simulink model "active_vehicle_controller_functions"  (R2020a)
settings: Solver=ode4  StartTime=0.0  StopTime=inf  FixedStep=1e-3  RelTol=1e-3
InitFcn:
  | clear mex
undefined symbols (not defined in the file or in its folder): DiscIntNeverNeededParam, vicrt_initcallback, vicrt_initmexcallback, vicrt_inputfile, vicrt_simulationmanager
libraries: simulink x1
(part 1 of 6)
settings Model: Creator=mcava  LastModifiedBy=lucas
settings DataIOCC: LimitDataPoints=on  SaveFormat=Array  SignalLoggingSaveFormat=ModelDataLogs  ReturnWorkspaceOutputs=off  SignalLoggingName=sigsOut
settings OptimizationCC: ExpressionDepthLimit=2147483647  InitFltsAndDblsToZero=on  LifeSpan=inf
settings DebuggingCC: SignalInfNanChecking=warning  SaveWithParameterizedLinksMsg=none  UnderspecifiedInitializationDetection=Classic  MergeDetectMultiDrivingBlocksExec=none  SignalResolutionControl=TryResolveAllWithWarning  MultiTaskDSMMsg=warning  MultiTaskCondExecSysMsg=none  FcnCallInpInsideContextMsg=warning  StateNameClashWarn=warning  SFUnexpectedBacktrackingDiag=warning  SFNoUnconditionalDefaultTransitionDiag=warning  SFExecutionAtInitializationDiag=none  ArithmeticOperatorsInVariantConditions=warning
settings HardwareCC: ProdBitPerPointer=32  ProdBitPerSizeT=32  ProdBitPerPtrDiffT=32  ProdLargestAtomicFloat=None  ProdIntDivRoundTo=Undefined  ProdEndianess=Unspecified  ProdWordSize=32  ProdHWDeviceType=32-bit Generic  TargetBitPerPointer=64  TargetBitPerSizeT=64  TargetBitPerPtrDiffT=64  TargetLongLongMode=on  TargetIntDivRoundTo=Zero  TargetEndianess=LittleEndian  TargetWordSize=64  TargetHWDeviceType=MATLAB Host  ProdEqTarget=off
settings ModelReferenceCC: PropagateSignalLabelsOutOfModel=off
settings SFSimCC: SimUseLocalCustomCode=off  SimParseCustomCode=off  CustomCodeUndefinedFunction=UseInterfaceOnly
settings RTWCC: RTWVerbose=off  RTWUseLocalCustomCode=off
settings CodeAppCC: GenerateComments=off  SimulinkBlockComments=off
settings GRTTargetCC: TargetFcnLib=ansi_tfl_tmw.mat  TargetLangStandard=C89/C90 (ANSI)  CombineOutputUpdateFcns=off  GRTInterface=on
settings ConfigComp: CovMetricSettings=dw  CovHtmlReporting=on  CovSaveCumulativeToWorkspaceVar=on  CovSaveSingleToWorkspaceVar=on  CovExternalEMLEnable=off

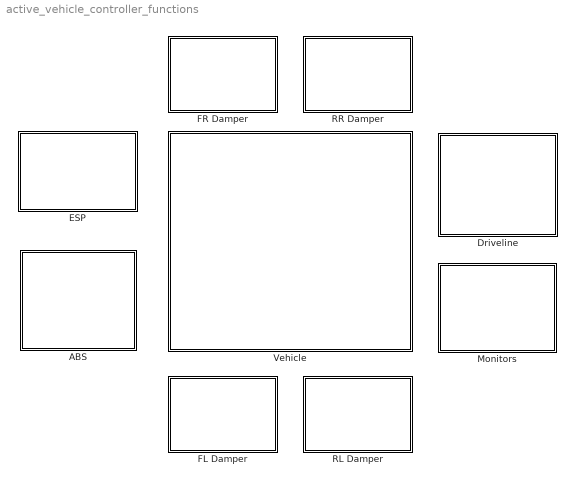
== system active_vehicle_controller_functions ==
  ABS : Subsystem  mask{ABSActive=on}
      mask prompts: ABSActive "Active"
      mask Display: image(imread('abs.jpg'))
  Driveline : Subsystem
      mask Display: image(imread('driveline.jpg'))
  ESP : Subsystem  mask(ESP Controller){ESPActive=on, WheelBase=2.838, SteeringRatio=(7.85/54)}
      mask prompts: ESPActive "Active"
      mask help:
      | Active toggle switches ESP On/Off
      | WheelBase and SteeringRatio parameters are used  to calculate theorical Vehicle Yaw Rate.
      mask Display: image(imread('esp.jpg'))
  FL Damper : Subsystem  mask{FLDamperActive=off}
      mask prompts: FLDamperActive "Active"
      mask Display: image(imread('damper.jpg'))
  FR Damper : Subsystem  mask{FRDamperActive=off}
      mask prompts: FRDamperActive "Active"
      mask Display: image(imread('damper.jpg'))
  Monitors : Subsystem
      mask Display: image(imread('monitors.jpg'))
  RL Damper : Subsystem  mask{RLDamperActive=off}
      mask prompts: RLDamperActive "Active"
      mask Display: image(imread('damper.jpg'))
  RR Damper : Subsystem  mask{RRDamperActive=off}
      mask prompts: RRDamperActive "Active"
      mask Display: image(imread('damper.jpg'))
  Vehicle : Subsystem
      mask Display: image(imread('vehicle.jpg'))

== system active_vehicle_controller_functions/ABS ==
  1st Order Lag L1 : TransferFcn  Denominator="[0.05  1]"
  1st Order Lag L2 : TransferFcn  Denominator="[0.05  1]"
  1st Order Lag R1 : TransferFcn  Denominator="[0.05  1]"
  1st Order Lag R2 : TransferFcn  Denominator="[0.05  1]"
  Brakes Already On? : Switch  Criteria=u2 > Threshold  SaturateOnIntegerOverflow=on
  Brakes Off : Constant  Value=0
  Brakes On : Constant
  Constant : Constant  Value=ABSActive
  Control Modes : Scope
  Demux : Demux
      settings: DisplayOption=none
  Memory : Memory  InitialCondition=[1,1,1,1]
  Mux : Mux
  NO ABS : Constant  Value=[1,1,1,1]
  Slip < Slip On? : Switch  Threshold=0.1  SaturateOnIntegerOverflow=on
  Slip > Slip Off? : Switch  Criteria=u2 > Threshold  Threshold=0.2  SaturateOnIntegerOverflow=on
  Slip Ratios : Product  Inputs=*/  SaturateOnIntegerOverflow=on  OutDataTypeStr=Inherit: Same as first input
  Slips : Scope
  Sum : Sum  Inputs=-+  SaturateOnIntegerOverflow=on  OutDataTypeStr=Inherit: Same as first input
  Vx > Vmin? : Switch  Criteria=u2 > Threshold  Threshold=5  SaturateOnIntegerOverflow=on
  Vx > Vmin?1 : Switch  Criteria=u2 > Threshold  SaturateOnIntegerOverflow=on
  tag scope: BrakesPressureGains=global
  wires:
  Sum/1 -> Slip Ratios/1
  [SprungMassCGVx] -> Slip Ratios/2, Sum/2, Vx > Vmin?/2
  Vx > Vmin?/1 -> Memory/1, Control Modes/1, Demux/1
  Slip > Slip Off?/1 -> Vx > Vmin?/1
  Brakes On/1 -> Brakes Already On?/1, Vx > Vmin?/3, Slip < Slip On?/3
  Brakes Off/1 -> Slip > Slip Off?/1, Brakes Already On?/3
  Slip Ratios/1 -> Slips/1, Slip > Slip Off?/2, Slip < Slip On?/2
  Slip < Slip On?/1 -> Slip > Slip Off?/3
  Memory/1 -> Brakes Already On?/2
  Brakes Already On?/1 -> Slip < Slip On?/1
  Demux/4 -> 1st Order Lag R2/1
  Demux/3 -> 1st Order Lag R1/1
  Demux/2 -> 1st Order Lag L2/1
  Demux/1 -> 1st Order Lag L1/1
  1st Order Lag L1/1 -> Mux/1
  1st Order Lag L2/1 -> Mux/2
  1st Order Lag R1/1 -> Mux/3
  1st Order Lag R2/1 -> Mux/4
  Mux/1 -> Vx > Vmin?1/1
  [TireTreadVx] -> Sum/1
  Constant/1 -> Vx > Vmin?1/2
  Vx > Vmin?1/1 -> [BrakesPressureGains]
  NO ABS/1 -> Vx > Vmin?1/3

== system active_vehicle_controller_functions/Driveline ==
  Clutch : Subsystem  mask{UserClutchActive=off}
      mask prompts: UserClutchActive "Active"
      mask Display: image(imread('clutch.jpg'))
  Engine : Subsystem  mask{UserEngineActive=off}
      mask prompts: UserEngineActive "Active"
      mask Display: image(imread('engine.jpg'))
  GearBox : Subsystem  mask{UserGearBoxActive=off}
      mask prompts: UserGearBoxActive "Active"
      mask Display: image(imread('gearbox.jpg'))
  Rear Differential : Subsystem  mask{RearDifferentialActive=off, DriveRatio=3.7}
      mask prompts: RearDifferentialActive "Active"; DriveRatio "Drive Ratio"
      mask Display: image(imread('differential.jpg'))

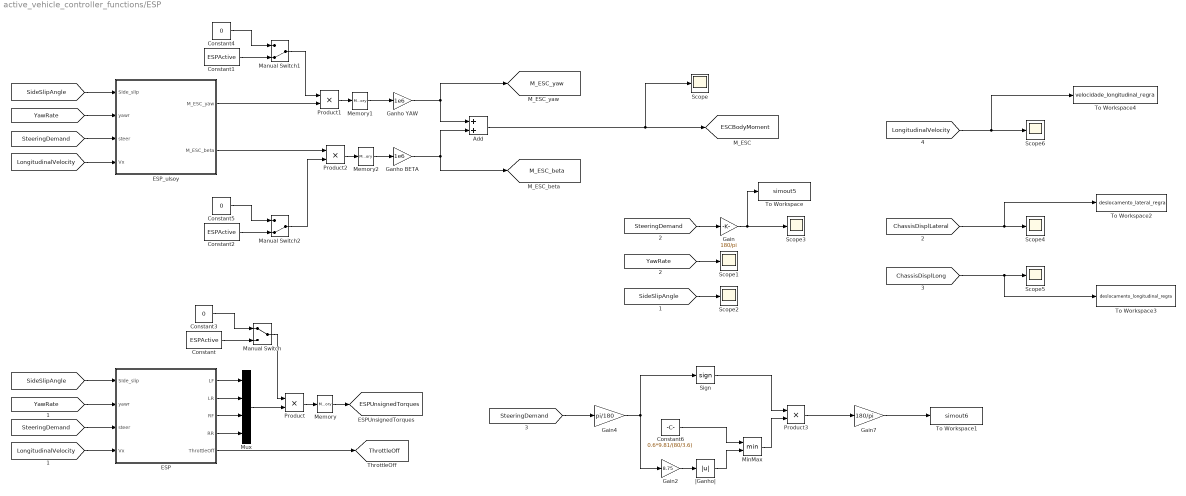
== system active_vehicle_controller_functions/ESP ==
  Add : Sum
  Constant : Constant  Value=ESPActive
  Constant1 : Constant  Value=ESPActive
  Constant2 : Constant  Value=ESPActive
  Constant3 : Constant  Value=0
  Constant4 : Constant  Value=0
  Constant5 : Constant  Value=0
  Constant6 : Constant  Value=0.6*9.81/(80/3.6)
  ESP : Subsystem  TreatAsAtomicUnit=on
  ESP_ulsoy : Subsystem  TreatAsAtomicUnit=on
  Gain : Gain  Gain=180/pi
  Gain2 : Gain  Gain=8.75
  Gain4 : Gain  Gain=pi/180
  Gain7 : Gain  Gain=180/pi
  Ganho BETA : Gain  Gain=1e6
  Ganho YAW : Gain  Gain=1e6
  Manual Switch : ManualSwitch
  Manual Switch1 : ManualSwitch  CurrentSetting=0
  Manual Switch2 : ManualSwitch  CurrentSetting=0
  Memory : Memory  InitialCondition=[0,0,0,0]
  Memory1 : Memory  InitialCondition=[0]
  Memory2 : Memory  InitialCondition=[0]
  MinMax : MinMax  Inputs=2
  Mux : Mux
  Product : Product  RndMeth=Zero  OutDataTypeStr=Inherit: Same as first input
  Product1 : Product  RndMeth=Zero  OutDataTypeStr=Inherit: Same as first input
  Product2 : Product  RndMeth=Zero  OutDataTypeStr=Inherit: Same as first input
  Product3 : Product
  Scope{,1..6} (7 alike) : Scope
  Sign : Signum
  To Workspace : ToWorkspace  VariableName=simout5  SaveFormat=Timeseries  SampleTime=-1
  To Workspace1 : ToWorkspace  VariableName=simout6  SaveFormat=Timeseries  SampleTime=-1
  To Workspace2 : ToWorkspace  VariableName=deslocamento_lateral_regra  SampleTime=-1
  To Workspace3 : ToWorkspace  VariableName=deslocamento_longitudinal_regra  SampleTime=-1
  To Workspace4 : ToWorkspace  VariableName=velocidade_longitudinal_regra  SaveFormat=Timeseries  SampleTime=-1
  |Ganho| : Abs
  tag scope: ESCBodyMoment=global, ESPUnsignedTorques=global, M_ESC_beta=global, M_ESC_yaw=global, ThrottleOff=global
  wires:
  [SideSlipAngle] -> ESP_ulsoy/1(SIde_slip)
  [LongitudinalVelocity] -> ESP_ulsoy/4(Vx)
  [YawRate] -> ESP_ulsoy/2("yawr ")
  [SteeringDemand] -> ESP_ulsoy/3(steer)
  Product1/1 -> Memory1/1
  Memory1/1 -> Ganho YAW/1
  ESP_ulsoy/1(M_ESC_yaw) -> Product1/2
  ESP/1(LF) -> Mux/1
  Mux/1 -> Product/2
  Memory/1 -> [ESPUnsignedTorques]
  [SteeringDemand] -> ESP/3(steer)
  ESP/4(RR) -> Mux/4
  ESP/2(LR) -> Mux/2
  [LongitudinalVelocity] -> ESP/4(Vx)
  [SideSlipAngle] -> ESP/1(SIde_slip)
  ESP/5(ThrottleOff) -> [ThrottleOff]
  Product/1 -> Memory/1
  ESP/3(RF) -> Mux/3
  [YawRate] -> ESP/2("yawr ")
  Memory2/1 -> Ganho BETA/1
  Product2/1 -> Memory2/1
  ESP_ulsoy/2(M_ESC_beta) -> Product2/1
  Add/1 -> [ESCBodyMoment], Scope/1
  Ganho YAW/1 -> [M_ESC_yaw], Add/1
  Ganho BETA/1 -> [M_ESC_beta], Add/2
  Manual Switch/1 -> Product/1
  Constant/1 -> Manual Switch/2
  Constant3/1 -> Manual Switch/1
  Constant4/1 -> Manual Switch1/1
  Constant1/1 -> Manual Switch1/2
  Manual Switch1/1 -> Product1/1
  Constant5/1 -> Manual Switch2/1
  Constant2/1 -> Manual Switch2/2
  Manual Switch2/1 -> Product2/2
  [YawRate] -> Scope1/1
  [SideSlipAngle] -> Scope2/1
  [SteeringDemand] -> Gain/1
  Gain/1 -> Scope3/1, To Workspace/1
  Gain4/1 -> Gain2/1, Sign/1
  |Ganho|/1 -> MinMax/2
  MinMax/1 -> Product3/2
  Constant6/1 -> MinMax/1
  [SteeringDemand] -> Gain4/1
  Sign/1 -> Product3/1
  Gain2/1 -> |Ganho|/1
  Gain7/1 -> To Workspace1/1
  Product3/1 -> Gain7/1
  [ChassisDisplLong] -> To Workspace3/1, Scope5/1
  [ChassisDisplLateral] -> Scope4/1, To Workspace2/1
  [LongitudinalVelocity] -> Scope6/1, To Workspace4/1

== system active_vehicle_controller_functions/FL Damper ==
  "C " : Gain  Gain=4000  OutDataTypeStr=Inherit: Same as input  ParamDataTypeStr=Inherit: Same as input
  Constant : Constant  Value=FLDamperActive
  Data Type Conversion : DataTypeConversion
  DmpF Lookup : Lookup  InputValues=|  Table=|
      InputValues=|
      | [ -1.5800000e+000 -1.0200000e+000 -7.7000000e-001 -5.1000000e-001 -3.8000000e-001 -2.5000000e-001 -1.3000000e-001 -5.0000000e-002 -3.0000000e-002 -1.0000000e-002  0.0000000e+000  1.0000000e-002  3.0000000e-002  5.0000000e-002  1.3000000e-001  2.6000000e-001  3.8000000e-001  5.1000000e-001  7.8000000e-001  1.0400000e+000  1.6200000e+000	
      | ]
      Table=|
      | [ -3.2605700e+003 -2.6592520e+003 -2.3311553e+003 -1.9825529e+003 -1.7569865e+003 -1.5314201e+003 -1.2853477e+003 -8.9573310e+002 -7.0015000e+002 -3.9192000e+002  0.0000000e+000  1.7058070e+002  4.3715920e+002  6.6272540e+002  1.0113279e+003  1.4419546e+003  1.6470150e+003  1.7905570e+003  2.1107987e+003  2.4057380e+003  3.1155941e+003	
      | ]
  Gain : Gain  Gain=1.2  OutDataTypeStr=Inherit: Same as input  ParamDataTypeStr=Inherit: Same as input
  Lin/Spline switch : ManualSwitch
  Logical Operator : Logic  Operator=NOT  AllPortsSameDT=off  OutDataTypeStr=boolean
  Memory : Memory
  Minus1 : UnaryMinus
  Minus2 : UnaryMinus
  Product : Product  RndMeth=Zero  OutDataTypeStr=Inherit: Same as first input
  Product1 : Product  RndMeth=Zero  OutDataTypeStr=Inherit: Same as first input
  Vx Lookup : Lookup  InputValues=|  Table=|
      InputValues=|
      | [ -5e-2 -1e-2 -5e-3 0 5e-3 1e-2 5e-2
      | ]
      Table=|
      | [ 1 1 1 0.2 1 1 1
      | ]
  tag scope: FLDamperForce=global, InternalFLDamperActive=global
  wires:
  Product/1 -> [FLDamperForce]
  Memory/1 -> Product/1
  Lin/Spline switch/1 -> Memory/1
  [FLDamperVelocity] -> Minus2/1, "C "/1
  Minus2/1 -> DmpF Lookup/1
  DmpF Lookup/1 -> Minus1/1
  "C "/1 -> Lin/Spline switch/2
  Minus1/1 -> Product1/2
  Product1/1 -> Lin/Spline switch/1
  Vx Lookup/1 -> Gain/1
  Gain/1 -> Product1/1
  [VerticalVelocity] -> Vx Lookup/1
  Data Type Conversion/1 -> [InternalFLDamperActive]
  Constant/1 -> Product/2, Logical Operator/1
  Logical Operator/1 -> Data Type Conversion/1

== system active_vehicle_controller_functions/FR Damper ==
  "C " : Gain  Gain=4000  OutDataTypeStr=Inherit: Same as input  ParamDataTypeStr=Inherit: Same as input
  Constant : Constant  Value=FRDamperActive
  Data Type Conversion : DataTypeConversion
  DmpF Lookup : Lookup  InputValues=|  Table=|
      InputValues=|
      | [ -1.5800000e+000 -1.0200000e+000 -7.7000000e-001 -5.1000000e-001 -3.8000000e-001 -2.5000000e-001 -1.3000000e-001 -5.0000000e-002 -3.0000000e-002 -1.0000000e-002  0.0000000e+000  1.0000000e-002  3.0000000e-002  5.0000000e-002  1.3000000e-001  2.6000000e-001  3.8000000e-001  5.1000000e-001  7.8000000e-001  1.0400000e+000  1.6200000e+000	
      | ]
      Table=|
      | [ -3.2605700e+003 -2.6592520e+003 -2.3311553e+003 -1.9825529e+003 -1.7569865e+003 -1.5314201e+003 -1.2853477e+003 -8.9573310e+002 -7.0015000e+002 -3.9192000e+002  0.0000000e+000  1.7058070e+002  4.3715920e+002  6.6272540e+002  1.0113279e+003  1.4419546e+003  1.6470150e+003  1.7905570e+003  2.1107987e+003  2.4057380e+003  3.1155941e+003	
      | ]
  Gain : Gain  Gain=1.2  OutDataTypeStr=Inherit: Same as input  ParamDataTypeStr=Inherit: Same as input
  Lin/Spline switch : ManualSwitch
  Logical Operator : Logic  Operator=NOT  AllPortsSameDT=off  OutDataTypeStr=boolean
  Memory : Memory
  Minus1 : UnaryMinus
  Minus2 : UnaryMinus
  Product : Product  RndMeth=Zero  OutDataTypeStr=Inherit: Same as first input
  Product1 : Product  RndMeth=Zero  OutDataTypeStr=Inherit: Same as first input
  Vx Lookup : Lookup  InputValues=|  Table=|
      InputValues=|
      | [ -5e-2 -1e-2 -5e-3 0 5e-3 1e-2 5e-2
      | ]
      Table=|
      | [ 1 1 1 0.2 1 1 1
      | ]
  tag scope: FRDamperForce=global, InternalFRDamperActive=global
  wires:
  Data Type Conversion/1 -> [InternalFRDamperActive]
  Memory/1 -> Product/1
  Product/1 -> [FRDamperForce]
  Lin/Spline switch/1 -> Memory/1
  [FRDamperVelocity] -> Minus2/1, "C "/1
  Minus2/1 -> DmpF Lookup/1
  DmpF Lookup/1 -> Minus1/1
  "C "/1 -> Lin/Spline switch/2
  Minus1/1 -> Product1/2
  Product1/1 -> Lin/Spline switch/1
  Vx Lookup/1 -> Gain/1
  Gain/1 -> Product1/1
  [VerticalVelocity] -> Vx Lookup/1
  Constant/1 -> Product/2, Logical Operator/1
  Logical Operator/1 -> Data Type Conversion/1

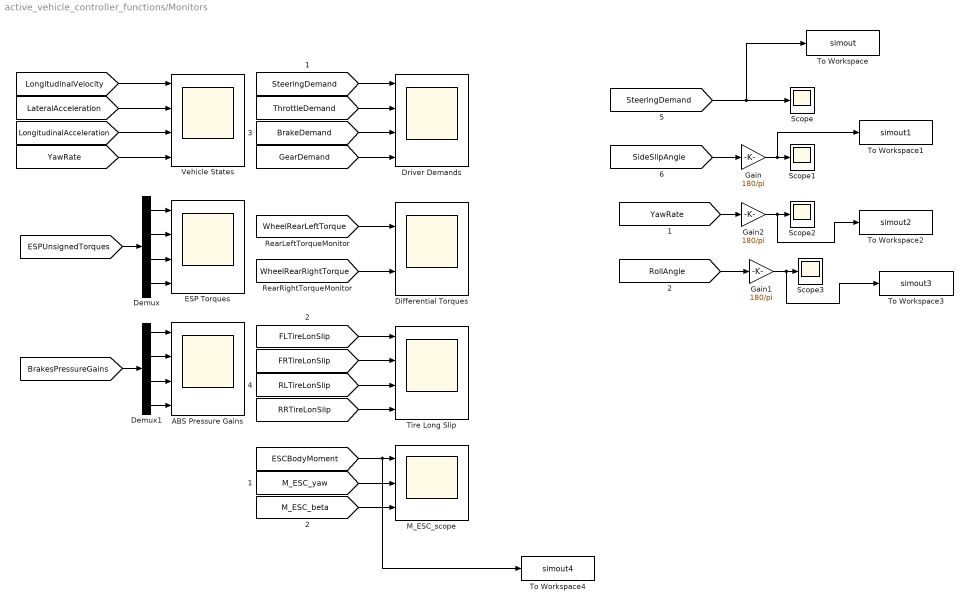
== system active_vehicle_controller_functions/Monitors ==
  ABS Pressure Gains : Scope  NumInputPorts=4
  Demux : Demux
  Demux1 : Demux
  Differential Torques : Scope  NumInputPorts=2
  Driver Demands : Scope  NumInputPorts=4
  ESP Torques : Scope  NumInputPorts=4
  Gain : Gain  Gain=180/pi
  Gain1 : Gain  Gain=180/pi
  Gain2 : Gain  Gain=180/pi
  M_ESC_scope : Scope  NumInputPorts=3
  Scope{,1..3} (4 alike) : Scope
  Tire Long Slip : Scope  NumInputPorts=4
  To Workspace : ToWorkspace  VariableName=simout  SaveFormat=Timeseries  SampleTime=-1
  To Workspace1 : ToWorkspace  VariableName=simout1  SaveFormat=Timeseries  SampleTime=-1
  To Workspace2 : ToWorkspace  VariableName=simout2  SaveFormat=Timeseries  SampleTime=-1
  To Workspace3 : ToWorkspace  VariableName=simout3  SaveFormat=Timeseries  SampleTime=-1
  To Workspace4 : ToWorkspace  VariableName=simout4  SaveFormat=Timeseries  SampleTime=-1
  Vehicle States : Scope  NumInputPorts=4
  wires:
  [LongitudinalVelocity] -> Vehicle States/1
  [LateralAcceleration] -> Vehicle States/2
  [LongitudinalAcceleration] -> Vehicle States/3
  [YawRate] -> Vehicle States/4
  [SteeringDemand] -> Driver Demands/1
  [ThrottleDemand] -> Driver Demands/2
  [BrakeDemand] -> Driver Demands/3
  [GearDemand] -> Driver Demands/4
  [ESPUnsignedTorques] -> Demux/1
  Demux/1 -> ESP Torques/1
  Demux/2 -> ESP Torques/2
  Demux/3 -> ESP Torques/3
  Demux/4 -> ESP Torques/4
  Demux1/1 -> ABS Pressure Gains/1
  Demux1/2 -> ABS Pressure Gains/2
  Demux1/3 -> ABS Pressure Gains/3
  Demux1/4 -> ABS Pressure Gains/4
  [BrakesPressureGains] -> Demux1/1
  [FLTireLonSlip] -> Tire Long Slip/1
  [FRTireLonSlip] -> Tire Long Slip/2
  [RLTireLonSlip] -> Tire Long Slip/3
  [RRTireLonSlip] -> Tire Long Slip/4
  [WheelRearLeftTorque] -> Differential Torques/1
  [WheelRearRightTorque] -> Differential Torques/2
  [ESCBodyMoment] -> To Workspace4/1, M_ESC_scope/1
  [M_ESC_yaw] -> M_ESC_scope/2
  [M_ESC_beta] -> M_ESC_scope/3
  [SteeringDemand] -> Scope/1, To Workspace/1
  [RollAngle] -> Gain1/1
  Gain1/1 -> To Workspace3/1, Scope3/1
  [YawRate] -> Gain2/1
  Gain2/1 -> To Workspace2/1, Scope2/1
  Gain/1 -> To Workspace1/1, Scope1/1
  [SideSlipAngle] -> Gain/1

== system active_vehicle_controller_functions/RL Damper ==
  "C " : Gain  Gain=4000  OutDataTypeStr=Inherit: Same as input  ParamDataTypeStr=Inherit: Same as input
  Constant : Constant  Value=RLDamperActive
  Data Type Conversion : DataTypeConversion
  DmpF Lookup : Lookup  InputValues=|  Table=|
      InputValues=|
      | [ -1.5800000e+000 -1.0200000e+000 -7.7000000e-001 -5.1000000e-001 -3.8000000e-001 -2.5000000e-001 -1.3000000e-001 -5.0000000e-002 -3.0000000e-002 -1.0000000e-002  0.0000000e+000  1.0000000e-002  3.0000000e-002  5.0000000e-002  1.3000000e-001  2.6000000e-001  3.8000000e-001  5.1000000e-001  7.8000000e-001  1.0400000e+000  1.6200000e+000	
      | ]
      Table=|
      | [ -3.2605700e+003 -2.6592520e+003 -2.3311553e+003 -1.9825529e+003 -1.7569865e+003 -1.5314201e+003 -1.2853477e+003 -8.9573310e+002 -7.0015000e+002 -3.9192000e+002  0.0000000e+000  1.7058070e+002  4.3715920e+002  6.6272540e+002  1.0113279e+003  1.4419546e+003  1.6470150e+003  1.7905570e+003  2.1107987e+003  2.4057380e+003  3.1155941e+003	
      | ]
  Gain : Gain  Gain=1.2  OutDataTypeStr=Inherit: Same as input  ParamDataTypeStr=Inherit: Same as input
  Lin/Spline switch : ManualSwitch
  Logical Operator : Logic  Operator=NOT  AllPortsSameDT=off  OutDataTypeStr=boolean
  Memory : Memory
  Minus1 : UnaryMinus
  Minus2 : UnaryMinus
  Product1 : Product  RndMeth=Zero  OutDataTypeStr=Inherit: Same as first input
  Product2 : Product  RndMeth=Zero  OutDataTypeStr=Inherit: Same as first input
  Scope : Scope
  Vx Lookup : Lookup  InputValues=|  Table=|
      InputValues=|
      | [ -5e-2 -1e-2 -5e-3 0 5e-3 1e-2 5e-2
      | ]
      Table=|
      | [ 1 1 1 0.2 1 1 1
      | ]
  tag scope: InternalRLDamperActive=global, RLDamperForce=global
  wires:
  Memory/1 -> Product2/1
  Product2/1 -> [RLDamperForce], Scope/1
  [RLDamperVelocity] -> Minus2/1, "C "/1
  Minus2/1 -> DmpF Lookup/1
  DmpF Lookup/1 -> Minus1/1
  "C "/1 -> Lin/Spline switch/2
  Lin/Spline switch/1 -> Memory/1
  Minus1/1 -> Product1/2
  Product1/1 -> Lin/Spline switch/1
  Vx Lookup/1 -> Gain/1
  Gain/1 -> Product1/1
  [VerticalVelocity] -> Vx Lookup/1
  Data Type Conversion/1 -> [InternalRLDamperActive]
  Constant/1 -> Product2/2, Logical Operator/1
  Logical Operator/1 -> Data Type Conversion/1

== system active_vehicle_controller_functions/RR Damper ==
  "C " : Gain  Gain=4000  OutDataTypeStr=Inherit: Same as input  ParamDataTypeStr=Inherit: Same as input
  Constant : Constant  Value=RRDamperActive
  Data Type Conversion : DataTypeConversion
  DmpF Lookup : Lookup  InputValues=|  Table=|
      InputValues=|
      | [ -1.5800000e+000 -1.0200000e+000 -7.7000000e-001 -5.1000000e-001 -3.8000000e-001 -2.5000000e-001 -1.3000000e-001 -5.0000000e-002 -3.0000000e-002 -1.0000000e-002  0.0000000e+000  1.0000000e-002  3.0000000e-002  5.0000000e-002  1.3000000e-001  2.6000000e-001  3.8000000e-001  5.1000000e-001  7.8000000e-001  1.0400000e+000  1.6200000e+000	
      | ]
      Table=|
      | [ -3.2605700e+003 -2.6592520e+003 -2.3311553e+003 -1.9825529e+003 -1.7569865e+003 -1.5314201e+003 -1.2853477e+003 -8.9573310e+002 -7.0015000e+002 -3.9192000e+002  0.0000000e+000  1.7058070e+002  4.3715920e+002  6.6272540e+002  1.0113279e+003  1.4419546e+003  1.6470150e+003  1.7905570e+003  2.1107987e+003  2.4057380e+003  3.1155941e+003	
      | ]
  Gain : Gain  Gain=1.2  OutDataTypeStr=Inherit: Same as input  ParamDataTypeStr=Inherit: Same as input
  Lin/Spline switch : ManualSwitch
  Logical Operator : Logic  Operator=NOT  AllPortsSameDT=off  OutDataTypeStr=boolean
  Memory1 : Memory
  Minus1 : UnaryMinus
  Minus2 : UnaryMinus
  Product : Product  RndMeth=Zero  OutDataTypeStr=Inherit: Same as first input
  Product1 : Product  RndMeth=Zero  OutDataTypeStr=Inherit: Same as first input
  Vx Lookup : Lookup  InputValues=|  Table=|
      InputValues=|
      | [ -5e-2 -1e-2 -5e-3 0 5e-3 1e-2 5e-2
      | ]
      Table=|
      | [ 1 1 1 0.2 1 1 1
      | ]
  tag scope: InternalRRDamperActive=global, RRDamperForce=global
  wires:
  Product/1 -> [RRDamperForce]
  Memory1/1 -> Product/1
  Lin/Spline switch/1 -> Memory1/1
  [VerticalVelocity] -> Vx Lookup/1
  Gain/1 -> Product1/1
  Vx Lookup/1 -> Gain/1
  Product1/1 -> Lin/Spline switch/1
  Minus1/1 -> Product1/2
  "C "/1 -> Lin/Spline switch/2
  DmpF Lookup/1 -> Minus1/1
  Minus2/1 -> DmpF Lookup/1
  [RRDamperVelocity] -> Minus2/1, "C "/1
  Data Type Conversion/1 -> [InternalRRDamperActive]
  Constant/1 -> Product/2, Logical Operator/1
  Logical Operator/1 -> Data Type Conversion/1

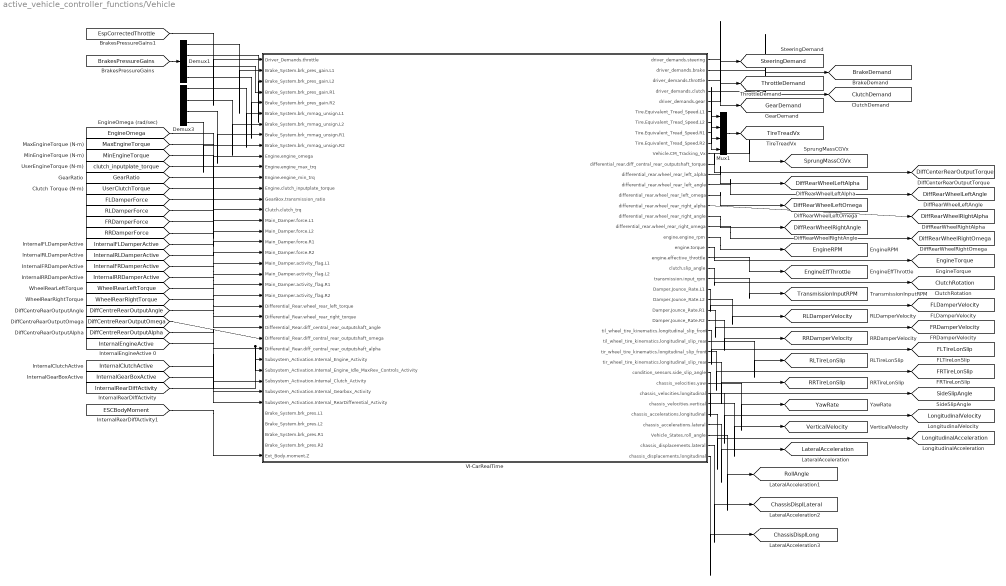
== system active_vehicle_controller_functions/Vehicle ==
  Demux1 : Demux
  Demux3 : Demux
  Mux1 : Mux
  VI-CarRealTime : Subsystem  InitFcn=vicrt_simulationmanager(0);  TreatAsAtomicUnit=on
      mask help: Full VI-CarRealTime mex integrated with IO Bus
      settings: CopyFcn=set_param(gcb, 'LinkStatus', 'none');  ModelCloseFcn=vicrt_simulationmanager(2);  OpenFcn=vicrt_simulationmanager(1);
      mask Display: image(imread('vehicle.jpg'));color('red');port_label('input',1,'Driver_Demands.throttle');port_label('input',2,'Brake_System.brk_pres_gain.L1');port_label('input',3,'Brake_System.brk_pres_gain.L2');port_label('input',4,'Brake_System.brk_pres_gain.R1');port_label('input',5,'Brake_System.brk_pres_gain.R2');port_label('input',6,'Brake_System.brk_mmag_unsign.L1');port_label('input',7,'Brake_System.brk_mmag_unsign.L2');port_label('input',8,'Brake_System.brk_mmag_unsign.R1');port_label('input',9,'Brake_System.brk_mmag_unsign.R2');port_label('input',10,'Engine.engine_omega');port_label('input',11,'Engine.engine_max_trq');port_label('input',12,'Engine.engine_min_trq');port_label('input',13,'Engine.clutch_inputplate_torque');port_label('input',14,'GearBox.transmission_ratio');port_label('input',15,'Clutch.clutch_trq');port_label('input',16,'Main_Damper.force.L1');port_label('input',17,'Main_Damper.force.L2');port_label('input',18,'Main_Damper.force.R1');port_label('input',19,'Main_Damper.force.R2');port_label('input',20,'Main_Damper.activity_flag.L1');port_label('input',21,'Main_Damper.activity_flag.L2');port_label('input',22,'Main_Damper.activity_flag.R1');port_label('input',23,'Main_Damper.activity_flag.R2');port_label('input',24,'Differential_Rear.wheel_rear_left_torque');port_label('input',25,'Differential_Rear.wheel_rear_right_torque');port_label('input',26,'Differential_Rear.diff_central_rear_outputshaft_angle');port_label('input',27,'Differential_Rear.diff_central_rear_outputshaft_omega');port_label('input',28,'Differential_Rear.diff_central_rear_outputshaft_alpha');port_label('input',29,'Subsystem_Activation.Internal_Engine_Activity');port_label('input',30,'Subsystem_Activation.Internal_Engine_Idle_MaxRev_Controls_Activity');port_label('input',31,'Subsystem_Activation.Internal_Clutch_Activity');port_label('input',32,'Subsystem_Activation.Internal_Gearbox_Activity');port_label('input',33,'Subsystem_Activation.Internal_RearDifferential_Activity');port_label('input',34,'Brake_System.brk_pres.L1');port_label('input',35,'Brake_System.brk_pres.L2');port_label('input',36,'Brake_System.brk_pres.R1');port_label('input',37,'Brake_System.brk_pres.R2');port_label('input',38,'Ext_Body.moment.Z');port_label('output',1,'driver_demands.steering');port_label('output',2,'driver_demands.brake');port_label('output',3,'driver_demands.throttle');port_label('output',4,'driver_demands.clutch');port_label('output',5,'driver_demands.gear');port_label('output',6,'Tire.Equivalent_Tread_Speed.L1');port_label('output',7,'Tire.Equivalent_Tread_Speed.L2');port_label('output',8,'Tire.Equivalent_Tread_Speed.R1');port_label('output',9,'Tire.Equivalent_Tread_Speed.R2');port_label('output',10,'Vehicle.CM_Tracking_Vx');port_label('output',11,'differential_rear.diff_central_rear_outputshaft_torque');port_label('output',12,'differential_rear.wheel_rear_left_alpha');port_label('output',13,'differential_rear.wheel_rear_left_angle');port_label('output',14,'differential_rear.wheel_rear_left_omega');port_label('output',15,'differential_rear.wheel_rear_right_alpha');port_label('output',16,'differential_rear.wheel_rear_right_angle');port_label('output',17,'differential_rear.wheel_rear_right_omega');port_label('output',18,'engine.engine_rpm');port_label('output',19,'engine.torque');port_label('output',20,'engine.effective_throttle');port_label('output',21,'clutch.slip_angle');port_label('output',22,'transmission.input_rpm');port_label('output',23,'Damper.Jounce_Rate.L1');port_label('output',24,'Damper.Jounce_Rate.L2');port_label('output',25,'Damper.Jounce_Rate.R1');port_label('output',26,'Damper.Jounce_Rate.R2');port_label('output',27,'til_wheel_tire_kinematics.longitudinal_slip_front');port_label('output',28,'til_wheel_tire_kinematics.longitudinal_slip_rear');port_label('output',29,'tir_wheel_tire_kinematics.longitudinal_slip_front');port_label('output',30,'tir_wheel_tire_kinematics.longitudinal_slip_rear');port_label('output',31,'condition_sensors.side_slip_angle');port_label('output',32,'chassis_velocities.yaw');port_label('output',33,'chassis_velocities.longitudinal');port_label('output',34,'chassis_velocities.vertical');port_label('output',35,'chassis_accelerations.longitudinal');port_label('output',36,'chassis_accelerations.lateral');port_label('output',37,'Vehicle_States.roll_angle');port_label('output',38,'chassis_displacements.lateral');port_label('output',39,'chassis_displacements.longitudinal');
  tag scope: BrakeDemand=global, ChassisDisplLateral=global, ChassisDisplLong=global, ClutchDemand=global, ClutchRotation=global, DiffCenterRearOutputTorque=global, DiffRearWheelLeftAlpha=global, DiffRearWheelLeftAngle=global, DiffRearWheelLeftOmega=global, DiffRearWheelRightAlpha=global, DiffRearWheelRightAngle=global, DiffRearWheelRightOmega=global, EngineEffThrottle=global, EngineRPM=global, EngineTorque=global, FLDamperVelocity=global, FLTireLonSlip=global, FRDamperVelocity=global, FRTireLonSlip=global, GearDemand=global, LateralAcceleration=global, LongitudinalAcceleration=global, LongitudinalVelocity=global, RLDamperVelocity=global, RLTireLonSlip=global, RRDamperVelocity=global, RRTireLonSlip=global, RollAngle=global, SideSlipAngle=global, SprungMassCGVx=global, SteeringDemand=global, ThrottleDemand=global, TireTreadVx=global, TransmissionInputRPM=global, VerticalVelocity=global, YawRate=global
  wires:
  Mux1/1 -> [TireTreadVx]
  VI-CarRealTime/1(driver_demands.steering) -> [SteeringDemand]
  VI-CarRealTime/2(driver_demands.brake) -> [BrakeDemand]
  VI-CarRealTime/3(driver_demands.throttle) -> [ThrottleDemand]
  VI-CarRealTime/4(driver_demands.clutch) -> [ClutchDemand]
  VI-CarRealTime/5(driver_demands.gear) -> [GearDemand]
  VI-CarRealTime/6(Tire.Equivalent_Tread_Speed.L1) -> Mux1/1
  VI-CarRealTime/7(Tire.Equivalent_Tread_Speed.L2) -> Mux1/2
  VI-CarRealTime/8(Tire.Equivalent_Tread_Speed.R1) -> Mux1/3
  VI-CarRealTime/9(Tire.Equivalent_Tread_Speed.R2) -> Mux1/4
  VI-CarRealTime/10(Vehicle.CM_Tracking_Vx) -> [SprungMassCGVx]
  VI-CarRealTime/14(differential_rear.wheel_rear_left_omega) -> [DiffRearWheelLeftOmega]
  VI-CarRealTime/19(engine.torque) -> [EngineTorque]
  VI-CarRealTime/21(clutch.slip_angle) -> [ClutchRotation]
  VI-CarRealTime/22(transmission.input_rpm) -> [TransmissionInputRPM]
  VI-CarRealTime/23(Damper.Jounce_Rate.L1) -> [FLDamperVelocity]
  VI-CarRealTime/24(Damper.Jounce_Rate.L2) -> [RLDamperVelocity]
  VI-CarRealTime/25(Damper.Jounce_Rate.R1) -> [FRDamperVelocity]
  VI-CarRealTime/26(Damper.Jounce_Rate.R2) -> [RRDamperVelocity]
  VI-CarRealTime/31(condition_sensors.side_slip_angle) -> [SideSlipAngle]
  VI-CarRealTime/32(chassis_velocities.yaw) -> [YawRate]
  VI-CarRealTime/33(chassis_velocities.longitudinal) -> [LongitudinalVelocity]
  VI-CarRealTime/34(chassis_velocities.vertical) -> [VerticalVelocity]
  VI-CarRealTime/35(chassis_accelerations.longitudinal) -> [LongitudinalAcceleration]
  VI-CarRealTime/36(chassis_accelerations.lateral) -> [LateralAcceleration]
  [BrakesPressureGains] -> Demux1/1
  Demux1/1 -> VI-CarRealTime/2(Brake_System.brk_pres_gain.L1)
  Demux1/2 -> VI-CarRealTime/3(Brake_System.brk_pres_gain.L2)
  Demux1/3 -> VI-CarRealTime/4(Brake_System.brk_pres_gain.R1)
  Demux1/4 -> VI-CarRealTime/5(Brake_System.brk_pres_gain.R2)
  [WheelRearLeftTorque] -> VI-CarRealTime/24(Differential_Rear.wheel_rear_left_torque)
  [WheelRearRightTorque] -> VI-CarRealTime/25(Differential_Rear.wheel_rear_right_torque)
  [EngineOmega] -> VI-CarRealTime/10(Engine.engine_omega)
  [MaxEngineTorque] -> VI-CarRealTime/11(Engine.engine_max_trq)
  [MinEngineTorque] -> VI-CarRealTime/12(Engine.engine_min_trq)
  [clutch_inputplate_torque] -> VI-CarRealTime/13(Engine.clutch_inputplate_torque)
  [GearRatio] -> VI-CarRealTime/14(GearBox.transmission_ratio)
  [UserClutchTorque] -> VI-CarRealTime/15(Clutch.clutch_trq)
  [FLDamperForce] -> VI-CarRealTime/16(Main_Damper.force.L1)
  [RLDamperForce] -> VI-CarRealTime/17(Main_Damper.force.L2)
  [FRDamperForce] -> VI-CarRealTime/18(Main_Damper.force.R1)
  [RRDamperForce] -> VI-CarRealTime/19(Main_Damper.force.R2)
  VI-CarRealTime/17(differential_rear.wheel_rear_right_omega) -> [DiffRearWheelRightOmega]
  VI-CarRealTime/27(til_wheel_tire_kinematics.longitudinal_slip_front) -> [FLTireLonSlip]
  VI-CarRealTime/28(til_wheel_tire_kinematics.longitudinal_slip_rear) -> [RLTireLonSlip]
  VI-CarRealTime/29(tir_wheel_tire_kinematics.longitudinal_slip_front) -> [FRTireLonSlip]
  VI-CarRealTime/30(tir_wheel_tire_kinematics.longitudinal_slip_rear) -> [RRTireLonSlip]
  [InternalClutchActive] -> VI-CarRealTime/31(Subsystem_Activation.Internal_Clutch_Activity)
  [InternalGearBoxActive] -> VI-CarRealTime/32(Subsystem_Activation.Internal_Gearbox_Activity)
  Demux3/1 -> VI-CarRealTime/6(Brake_System.brk_mmag_unsign.L1)
  Demux3/2 -> VI-CarRealTime/7(Brake_System.brk_mmag_unsign.L2)
  Demux3/3 -> VI-CarRealTime/8(Brake_System.brk_mmag_unsign.R1)
  Demux3/4 -> VI-CarRealTime/9(Brake_System.brk_mmag_unsign.R2)
  [EspCorrectedThrottle] -> VI-CarRealTime/1(Driver_Demands.throttle)
  VI-CarRealTime/18(engine.engine_rpm) -> [EngineRPM]
  [InternalEngineActive] -> VI-CarRealTime/29(Subsystem_Activation.Internal_Engine_Activity), VI-CarRealTime/30(Subsystem_Activation.Internal_Engine_Idle_MaxRev_Controls_Activity)
  [InternalRearDiffActivity] -> VI-CarRealTime/33(Subsystem_Activation.Internal_RearDifferential_Activity)
  [DiffCentreRearOutputOmega] -> VI-CarRealTime/27(Differential_Rear.diff_central_rear_outputshaft_omega)
  [InternalRRDamperActive] -> VI-CarRealTime/23(Main_Damper.activity_flag.R2)
  [InternalFLDamperActive] -> VI-CarRealTime/20(Main_Damper.activity_flag.L1)
  [InternalRLDamperActive] -> VI-CarRealTime/21(Main_Damper.activity_flag.L2)
  [InternalFRDamperActive] -> VI-CarRealTime/22(Main_Damper.activity_flag.R1)
  VI-CarRealTime/20(engine.effective_throttle) -> [EngineEffThrottle]
  [DiffCentreRearOutputAngle] -> VI-CarRealTime/26(Differential_Rear.diff_central_rear_outputshaft_angle)
  [DiffCentreRearOutputAlpha] -> VI-CarRealTime/28(Differential_Rear.diff_central_rear_outputshaft_alpha)
  VI-CarRealTime/11(differential_rear.diff_central_rear_outputshaft_torque) -> [DiffCenterRearOutputTorque]
  VI-CarRealTime/12(differential_rear.wheel_rear_left_alpha) -> [DiffRearWheelLeftAlpha]
  VI-CarRealTime/13(differential_rear.wheel_rear_left_angle) -> [DiffRearWheelLeftAngle]
  VI-CarRealTime/15(differential_rear.wheel_rear_right_alpha) -> [DiffRearWheelRightAlpha]
  VI-CarRealTime/16(differential_rear.wheel_rear_right_angle) -> [DiffRearWheelRightAngle]
  [ESCBodyMoment] -> VI-CarRealTime/38(Ext_Body.moment.Z)
  VI-CarRealTime/37(Vehicle_States.roll_angle) -> [RollAngle]
  VI-CarRealTime/38(chassis_displacements.lateral) -> [ChassisDisplLateral]
  VI-CarRealTime/39(chassis_displacements.longitudinal) -> [ChassisDisplLong]

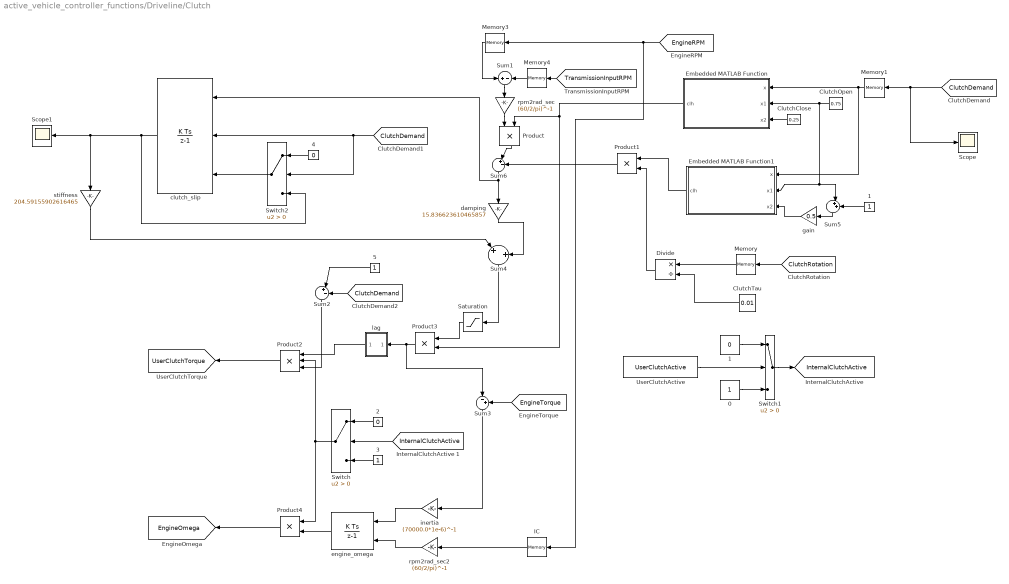
== system active_vehicle_controller_functions/Driveline/Clutch ==
  {0..1,3,5} (4 alike) : Constant
  "1 " : Constant  Value=0
  2 : Constant  Value=0
  4 : Constant  Value=0
  ClutchClose : Constant  Value=0.25
  ClutchOpen : Constant  Value=0.75
  ClutchTau : Constant  Value=0.01
  Divide : Product  Inputs=*/  OutDataTypeStr=Inherit: Same as first input
  Embedded MATLAB Function : MATLAB Function  TreatAsAtomicUnit=on
  Embedded MATLAB Function1 : MATLAB Function  TreatAsAtomicUnit=on
  IC : Memory  InitialCondition=6027  InheritSampleTime=on
  Memory : Memory
  Memory1 : Memory
  Memory3 : Memory  InitialCondition=6027  InheritSampleTime=on
  Memory4 : Memory  InitialCondition=6027  InheritSampleTime=on
  Product{,1,3..4} (4 alike) : Product  RndMeth=Zero  OutDataTypeStr=Inherit: Same as first input
  Product2 : Product  Inputs=3  RndMeth=Zero  OutDataTypeStr=Inherit: Same as first input
  Saturation : Saturate  UpperLimit=1000  LowerLimit=-1000
  Scope : Scope
  Scope1 : Scope
  Sum1 : Sum  Inputs=+-  OutDataTypeStr=Inherit: Same as first input
  Sum2 : Sum  Inputs=||+-  OutDataTypeStr=Inherit: Same as first input
  Sum3 : Sum  Inputs=|-+  OutDataTypeStr=Inherit: Same as first input
  Sum4 : Sum  Inputs=|+||+  OutDataTypeStr=Inherit: Same as first input
  Sum5 : Sum  Inputs=||++  OutDataTypeStr=Inherit: Same as first input
  Sum6 : Sum  Inputs=||+-  OutDataTypeStr=Inherit: Same as first input
  Switch : Switch  Criteria=u2 > Threshold
  Switch1 : Switch  Criteria=u2 > Threshold
  Switch2 : Switch  Criteria=u2 > Threshold
  UserClutchActive : Constant  Value=UserClutchActive
  clutch_slip : DiscreteIntegrator  ExternalReset=level  InitialConditionSource=external  SampleTime=-1  LowerSaturationLimit=-500  ICPrevOutput=DiscIntNeverNeededParam  ICPrevScaledInput=DiscIntNeverNeededParam
  damping : Gain  Gain=15.836623610465857  OutDataTypeStr=Inherit: Same as input  ParamDataTypeStr=Inherit: Same as input
  engine_omega : DiscreteIntegrator  InitialConditionSource=external  InitialCondition=600  SampleTime=-1  LowerSaturationLimit=1000/60*2*pi  ICPrevOutput=DiscIntNeverNeededParam  ICPrevScaledInput=DiscIntNeverNeededParam
  gain : Gain  Gain=0.5  OutDataTypeStr=Inherit: Same as input  ParamDataTypeStr=Inherit: Same as input
  inertia : Gain  Gain=(70000.0*1e-6)^-1  OutDataTypeStr=Inherit: Same as input  ParamDataTypeStr=Inherit: Same as input
  lag : Subsystem
  rpm2rad_sec : Gain  Gain=(60/2/pi)^-1  OutDataTypeStr=Inherit: Same as input  ParamDataTypeStr=Inherit: Same as input
  rpm2rad_sec2 : Gain  Gain=(60/2/pi)^-1  OutDataTypeStr=Inherit: Same as input  ParamDataTypeStr=Inherit: Same as input
  stiffness : Gain  Gain=204.59155902616465  OutDataTypeStr=Inherit: Same as input  ParamDataTypeStr=Inherit: Same as input
  tag scope: EngineOmega=global, InternalClutchActive=global, UserClutchTorque=global
  wires:
  [EngineRPM] -> Memory3/1, IC/1
  [TransmissionInputRPM] -> Memory4/1
  stiffness/1 -> Sum4/1
  damping/1 -> Sum4/2
  ClutchOpen/1 -> Embedded MATLAB Function/2(x1), Sum5/1, Embedded MATLAB Function1/2(x1)
  ClutchClose/1 -> Embedded MATLAB Function/3(x2)
  Embedded MATLAB Function/1(clh) -> Product/2, Product3/2
  Sum1/1 -> rpm2rad_sec/1
  1/1 -> Sum5/2
  Sum5/1 -> gain/1
  ClutchTau/1 -> Divide/2
  Divide/1 -> Product1/2
  Embedded MATLAB Function1/1(clh) -> Product1/1
  Product1/1 -> Sum6/2
  Sum6/1 -> damping/1, clutch_slip/1
  rpm2rad_sec/1 -> Product/1
  rpm2rad_sec2/1 -> engine_omega/2
  Product/1 -> Sum6/1
  Sum3/1 -> inertia/1
  inertia/1 -> engine_omega/1
  Memory/1 -> Divide/1
  Memory1/1 -> Embedded MATLAB Function1/1(x), Embedded MATLAB Function/1(x)
  gain/1 -> Embedded MATLAB Function1/3(x2)
  IC/1 -> rpm2rad_sec2/1
  Product3/1 -> Sum3/1, lag/1(In1)
  Memory3/1 -> Sum1/1
  Memory4/1 -> Sum1/2
  [ClutchRotation] -> Memory/1
  Saturation/1 -> Product3/1
  Sum4/1 -> Saturation/1
  Product2/1 -> [UserClutchTorque]
  Switch/1 -> Product2/2, Product4/1
  2/1 -> Switch/1
  [InternalClutchActive] -> Switch/2
  3/1 -> Switch/3
  engine_omega/1 -> Product4/2
  UserClutchActive/1 -> Switch1/2
  Switch1/1 -> [InternalClutchActive]
  "1 "/1 -> Switch1/1
  0/1 -> Switch1/3
  clutch_slip/1 -> Switch2/3, stiffness/1, Scope1/1
  [EngineTorque] -> Sum3/2
  Switch2/1 -> clutch_slip/3
  4/1 -> Switch2/1
  [ClutchDemand] -> Memory1/1, Scope/1
  lag/1(Out1) -> Product2/1
  Product4/1 -> [EngineOmega]
  5/1 -> Sum2/1
  Sum2/1 -> Product2/3
  [ClutchDemand] -> Switch2/2, clutch_slip/2
  [ClutchDemand] -> Sum2/2

== system active_vehicle_controller_functions/Driveline/Engine ==
  0 : Constant
  "1 " : Constant  Value=0
  Engine Maps : Subsystem
  Memory : Memory
  Product1 : Product  RndMeth=Zero  OutDataTypeStr=Inherit: Same as first input
  Product2 : Product  RndMeth=Zero  OutDataTypeStr=Inherit: Same as first input
  Sum : Sum  Inputs=+-  OutDataTypeStr=Inherit: Same as first input
  Switch1 : Switch  Criteria=u2 > Threshold
  ThrottleOff (from ESP) : Subsystem  mask{ThrottleOffScale=.1}
      mask prompts: ThrottleOffScale "Thottle Off Scale"
  UserEngineActive : Constant  Value=UserEngineActive
  tag scope: EspCorrectedThrottle=global, InternalEngineActive=global, MaxEngineTorque=global, MinEngineTorque=global, clutch_inputplate_torque=global
  wires:
  [EngineRPM] -> Engine Maps/1(RPM)
  [EngineEffThrottle] -> Memory/1
  Engine Maps/1(MaxEngineTorque) -> [MaxEngineTorque]
  Engine Maps/2(MinEngineTorque) -> [MinEngineTorque]
  Product1/1 -> Engine Maps/2(Throttle), Sum/1
  ThrottleOff (from ESP)/1(ThrottleGain) -> Product1/2
  Engine Maps/3(EngineTorque) -> [clutch_inputplate_torque]
  Sum/1 -> Product2/1
  [InternalEngineActive] -> Product2/2
  Product2/1 -> [EspCorrectedThrottle]
  Memory/1 -> Product1/1, Sum/2
  UserEngineActive/1 -> Switch1/2
  Switch1/1 -> [InternalEngineActive]
  "1 "/1 -> Switch1/1
  0/1 -> Switch1/3

== system active_vehicle_controller_functions/Driveline/GearBox ==
  " " : Memory
  0 : Constant
  "1 " : Constant  Value=0
  Gear Ratio : Lookup  InputValues=[1 2 3 4 5 6]  Table=[2.88 1.77 1.27 1.0 0.88 0.71]
  Switch : Switch  Criteria=u2 > Threshold
  UserGearBoxActive : Constant  Value=UserGearBoxActive
  tag scope: GearRatio=global, InternalGearBoxActive=global
  wires:
  [GearDemand] -> " "/1
  Gear Ratio/1 -> [GearRatio]
  " "/1 -> Gear Ratio/1
  UserGearBoxActive/1 -> Switch/2
  Switch/1 -> [InternalGearBoxActive]
  "1 "/1 -> Switch/1
  0/1 -> Switch/3

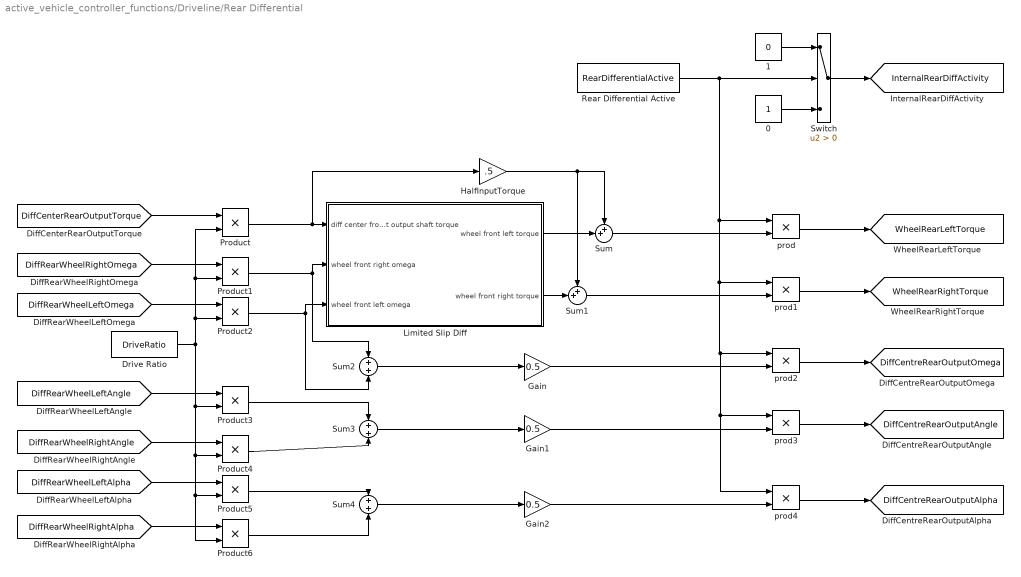
== system active_vehicle_controller_functions/Driveline/Rear Differential ==
  0 : Constant
  "1 " : Constant  Value=0
  Drive Ratio : Constant  Value=DriveRatio
  Gain : Gain  Gain=0.5
  Gain1 : Gain  Gain=0.5
  Gain2 : Gain  Gain=0.5
  HalfInputTorque : Gain  Gain=.5
  Limited Slip Diff : Subsystem  mask{C0=0, C1=.2, C2=1.05, C3=1.1}
  Product{,1..6} (7 alike) : Product
  Rear Differential Active : Constant  Value=RearDifferentialActive
  Sum : Sum  Inputs=++|
  Sum1 : Sum  Inputs=++|
  Sum2 : Sum
  Sum3 : Sum
  Sum4 : Sum
  Switch : Switch  Criteria=u2 > Threshold
  prod{,1..4} (5 alike) : Product
  tag scope: DiffCentreRearOutputAlpha=global, DiffCentreRearOutputAngle=global, DiffCentreRearOutputOmega=global, InternalRearDiffActivity=global, WheelRearLeftTorque=global, WheelRearRightTorque=global
  wires:
  [DiffRearWheelRightAngle] -> Product4/1
  [DiffRearWheelLeftAlpha] -> Product5/1
  [DiffRearWheelLeftAngle] -> Product3/1
  Sum2/1 -> Gain/1
  [DiffRearWheelRightOmega] -> Product1/1
  [DiffRearWheelLeftOmega] -> Product2/1
  [DiffCenterRearOutputTorque] -> Product/1
  HalfInputTorque/1 -> Sum/1, Sum1/1
  Sum3/1 -> Gain1/1
  [DiffRearWheelRightAlpha] -> Product6/1
  Sum4/1 -> Gain2/1
  Limited Slip Diff/1(wheel front left torque) -> Sum/2
  Limited Slip Diff/2(wheel front right torque) -> Sum1/2
  Product/1 -> Limited Slip Diff/1(diff center front output shaft torque), HalfInputTorque/1
  Product1/1 -> Limited Slip Diff/2(wheel front right omega), Sum2/1
  Product2/1 -> Limited Slip Diff/3(wheel front left omega), Sum2/2
  Product3/1 -> Sum3/1
  Product4/1 -> Sum3/2
  Product5/1 -> Sum4/1
  Product6/1 -> Sum4/2
  Drive Ratio/1 -> Product6/2, Product5/2, Product4/2, Product3/2, Product2/2, Product1/2, Product/2
  Rear Differential Active/1 -> Switch/2, prod4/1, prod3/1, prod2/1, prod1/1, prod/1
  Sum/1 -> prod/2
  Sum1/1 -> prod1/2
  Gain/1 -> prod2/2
  Gain1/1 -> prod3/2
  Gain2/1 -> prod4/2
  Switch/1 -> [InternalRearDiffActivity]
  "1 "/1 -> Switch/1
  0/1 -> Switch/3
  prod/1 -> [WheelRearLeftTorque]
  prod1/1 -> [WheelRearRightTorque]
  prod2/1 -> [DiffCentreRearOutputOmega]
  prod3/1 -> [DiffCentreRearOutputAngle]
  prod4/1 -> [DiffCentreRearOutputAlpha]

== system active_vehicle_controller_functions/ESP/ESP ==
  SIde_slip : Inport
  "yawr " : Inport  Port=2
  steer : Inport  Port=3
  Vx : Inport  Port=4
  Demux : Demux
  ESP Sensors : Scope  NumInputPorts=3
  Embedded MATLAB Function : MATLAB Function  TreatAsAtomicUnit=on
  Mux1 : Mux
  SteeringRatio : Constant  Value=SteeringRatio
  WheelBase : Constant  Value=WheelBase
  YawErrorToTorqueGain : Gain  Gain=[25 25 25 25]  OutDataTypeStr=Inherit: Same as input  ParamDataTypeStr=Inherit: Same as input
  LF : Outport  VectorParamsAs1DForOutWhenUnconnected=off
  LR : Outport  Port=2  VectorParamsAs1DForOutWhenUnconnected=off
  RF : Outport  Port=3  VectorParamsAs1DForOutWhenUnconnected=off
  RR : Outport  Port=4  VectorParamsAs1DForOutWhenUnconnected=off
  ThrottleOff : Outport  Port=5  VectorParamsAs1DForOutWhenUnconnected=off
  wires:
  Embedded MATLAB Function/7(yawrT) -> ESP Sensors/3
  Embedded MATLAB Function/5(overSteerRate) -> ESP Sensors/1
  YawErrorToTorqueGain/1 -> Demux/1
  Mux1/1 -> YawErrorToTorqueGain/1
  Embedded MATLAB Function/4(RR) -> Mux1/4
  Embedded MATLAB Function/3(RL) -> Mux1/3
  Embedded MATLAB Function/2(FR) -> Mux1/2
  Embedded MATLAB Function/1(FL) -> Mux1/1
  Demux/1 -> LF/1
  SIde_slip/1 -> Embedded MATLAB Function/1(SideSlip)
  Demux/2 -> RF/1
  Demux/3 -> LR/1
  steer/1 -> Embedded MATLAB Function/3(SWA)
  Demux/4 -> RR/1
  Vx/1 -> Embedded MATLAB Function/4(Vx)
  "yawr "/1 -> Embedded MATLAB Function/2(yawr)
  Embedded MATLAB Function/6(throttleOffTrigger) -> ThrottleOff/1, ESP Sensors/2
  WheelBase/1 -> Embedded MATLAB Function/5(WheelBase)
  SteeringRatio/1 -> Embedded MATLAB Function/6(steerRatio)

== system active_vehicle_controller_functions/ESP/ESP_ulsoy ==
  SIde_slip : Inport
  "yawr " : Inport  Port=2
  steer : Inport  Port=3
  Vx : Inport  Port=4
  Derivative : Derivative
  Embedded MATLAB Function : MATLAB Function  TreatAsAtomicUnit=on
  SteeringRatio : Constant  Value=SteeringRatio
  WheelBase : Constant  Value=WheelBase
  M_ESC_yaw : Outport  VectorParamsAs1DForOutWhenUnconnected=off
  M_ESC_beta : Outport  Port=2  VectorParamsAs1DForOutWhenUnconnected=off
  wires:
  SIde_slip/1 -> Derivative/1, Embedded MATLAB Function/1(SideSlip)
  steer/1 -> Embedded MATLAB Function/4(SWA)
  Vx/1 -> Embedded MATLAB Function/5(Vx)
  "yawr "/1 -> Embedded MATLAB Function/3(yawr)
  WheelBase/1 -> Embedded MATLAB Function/6(WheelBase)
  SteeringRatio/1 -> Embedded MATLAB Function/7(steerRatio)
  Embedded MATLAB Function/1(M_ESC_yaw) -> M_ESC_yaw/1
  Derivative/1 -> Embedded MATLAB Function/2(SideSlip_derivate)
  Embedded MATLAB Function/2(M_ESC_beta) -> M_ESC_beta/1
